simulink model "Lecture_1"  (R2025a)
settings: Solver=VariableStepAuto  StartTime=0.0  StopTime=t_f  RelTol=1e-3
values from neighbouring files (symbols this model uses):
  G_d = [1 0.12 1]    [Simulink_exercise_01.m]
  G_n = [1 1]    [Simulink_exercise_01.m]
  T_s = 0.01    [Simulink_exercise_01.m]
settings Model: Creator=Mads2  LastModifiedBy=Mads2

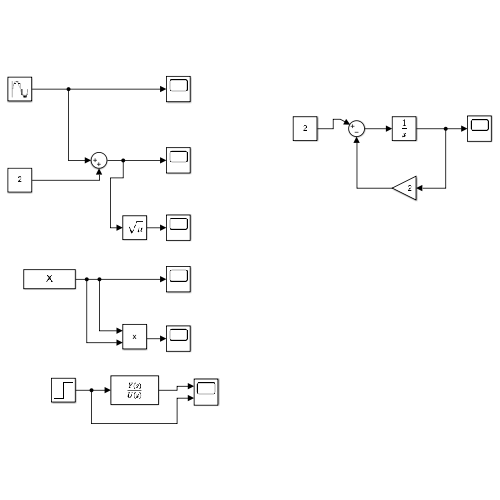
[thumbnail: Simulink's stored preview of the top-level diagram]
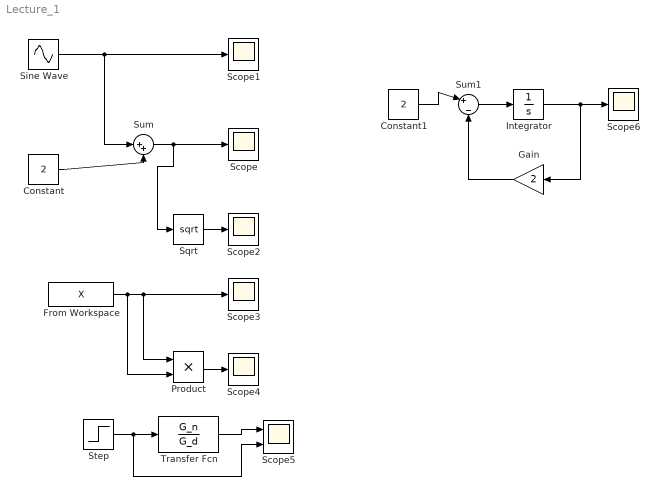
== system Lecture_1 ==
  Constant : Constant  Value=2
  Constant1 : Constant  Value=2
  From Workspace : FromWorkspace  VariableName=X  SampleTime=T_s
  Gain : Gain  Gain=2
  Integrator : Integrator
  Product : Product
  Scope{,1..4,6} (6 alike) : Scope
      Scope settings: ActiveDisplayYMinimum=-2.9645190145575797  ActiveDisplayYMaximum=4.3002244812227879
      Scope1 settings: ActiveDisplayYMinimum=-1.2499999834854445  ActiveDisplayYMaximum=1.2499999934801123
      Scope2 settings: ActiveDisplayYMinimum=-2.9645190145575797  ActiveDisplayYMaximum=4.3002244812227879  DataLoggingVariableName=ScopeData2
      Scope3 settings: ActiveDisplayYMinimum=-1.6119288457218386  ActiveDisplayYMaximum=10.221572799471177  DataLoggingVariableName=ScopeData3
      Scope4 settings: ActiveDisplayYMinimum=-6.3245616733942729  ActiveDisplayYMaximum=47.376336143719328  DataLoggingVariableName=ScopeData4
      Scope6 settings: DataLoggingVariableName=ScopeData6
  Scope5 : Scope  NumInputPorts=2
      settings: ActiveDisplayYMinimum=-1.7585839961347625  ActiveDisplayYMaximum=5.1602193331798718  DataLoggingVariableName=ScopeData5
  Sine Wave : Sin  SampleTime=T_s
  Sqrt : Sqrt
  Step : Step  SampleTime=0
  Sum : Sum  Inputs=|++
  Sum1 : Sum  Inputs=|+|-
  Transfer Fcn : TransferFcn  Numerator=G_n  Denominator=G_d
  wires:
  Constant/1 -> Sum/2
  Sum/1 -> Sqrt/1, Scope/1
  Sine Wave/1 -> Scope1/1, Sum/1
  Sqrt/1 -> Scope2/1
  From Workspace/1 -> Product/2, Scope3/1, Product/1
  Product/1 -> Scope4/1
  Transfer Fcn/1 -> Scope5/1
  Step/1 -> Scope5/2, Transfer Fcn/1
  Gain/1 -> Sum1/2
  Constant1/1 -> Sum1/1
  Sum1/1 -> Integrator/1
  Integrator/1 -> Scope6/1, Gain/1
